simulink model "tren_model"  (Simulink 7.1)
settings: Solver=ode45  StartTime=0.0  StopTime=10.0  RelTol=1e-3
values from neighbouring files (symbols this model uses):
  Ltr1y1 = 12.25    [train_katsayi.m]
  Ltr1y2 = 12.25    [train_katsayi.m]
  Ltr2y1 = 1.25    [train_katsayi.m]
  Ltr2y2 = 1.25    [train_katsayi.m]
  Ltr3y1 = 1.25    [train_katsayi.m]
  Ltr3y2 = 1.25    [train_katsayi.m]
  Vtr = 40    [train_katsayi.m]
settings Model: Creator=DOAN  LastModifiedBy=DOAN

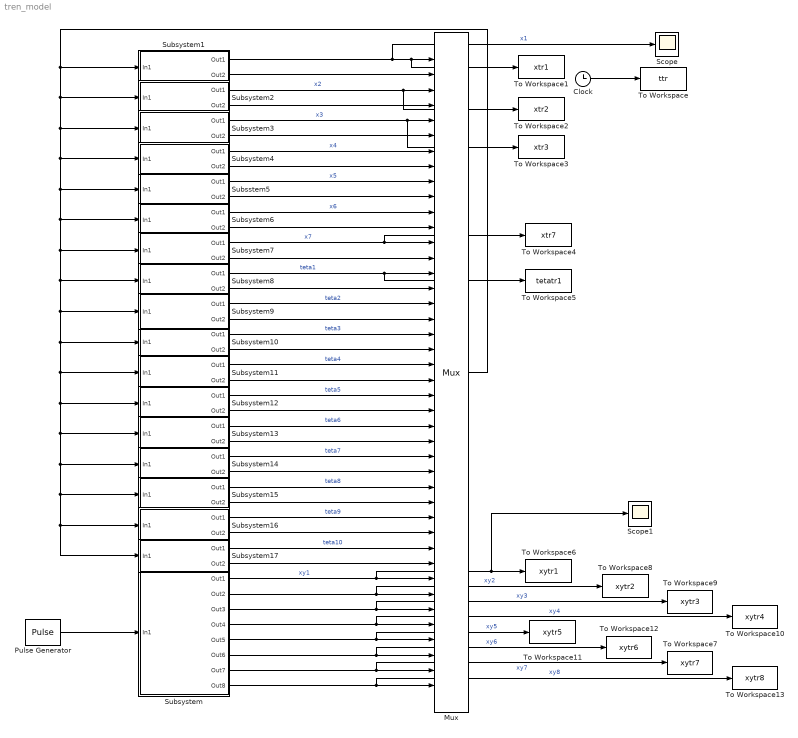
== system tren_model ==
  Clock : Clock
      settings: Decimation=10
  Mux : Mux  Inputs=42
  Pulse Generator : DiscretePulseGenerator  PulseType=Time based  Amplitude=-0.01  Period=0.5  PulseWidth=0.025
  Scope : Scope
      settings: TimeRange=10  YMin=-5e-006  YMax=1.000000000000001e-006
  Scope1 : Scope
      settings: TimeRange=10  YMin=-5e-006  YMax=1.000000000000001e-006
  Subsstem5 : Subsystem
  Subsystem : Subsystem
  Subsystem1 : Subsystem
  Subsystem10 : Subsystem
  Subsystem11 : Subsystem
  Subsystem12 : Subsystem
  Subsystem13 : Subsystem
  Subsystem14 : Subsystem
  Subsystem15 : Subsystem
  Subsystem16 : Subsystem
  Subsystem17 : Subsystem
  Subsystem2 : Subsystem
  Subsystem3 : Subsystem
  Subsystem4 : Subsystem
  Subsystem6 : Subsystem
  Subsystem7 : Subsystem
  Subsystem8 : Subsystem
  Subsystem9 : Subsystem
  To Workspace : ToWorkspace  VariableName=ttr  SampleTime=-1  SaveFormat=Array
  To Workspace1 : ToWorkspace  VariableName=xtr1  SampleTime=-1  SaveFormat=Array
  To Workspace10 : ToWorkspace  VariableName=xytr4  SampleTime=-1  SaveFormat=Array
  To Workspace11 : ToWorkspace  VariableName=xytr5  SampleTime=-1  SaveFormat=Array
  To Workspace12 : ToWorkspace  VariableName=xytr6  SampleTime=-1  SaveFormat=Array
  To Workspace13 : ToWorkspace  VariableName=xytr8  SampleTime=-1  SaveFormat=Array
  To Workspace2 : ToWorkspace  VariableName=xtr2  SampleTime=-1  SaveFormat=Array
  To Workspace3 : ToWorkspace  VariableName=xtr3  SampleTime=-1  SaveFormat=Array
  To Workspace4 : ToWorkspace  VariableName=xtr7  SampleTime=-1  SaveFormat=Array
  To Workspace5 : ToWorkspace  VariableName=tetatr1  SampleTime=-1  SaveFormat=Array
  To Workspace6 : ToWorkspace  VariableName=xytr1  SampleTime=-1  SaveFormat=Array
  To Workspace7 : ToWorkspace  VariableName=xytr7  SampleTime=-1  SaveFormat=Array
  To Workspace8 : ToWorkspace  VariableName=xytr2  SampleTime=-1  SaveFormat=Array
  To Workspace9 : ToWorkspace  VariableName=xytr3  SampleTime=-1  SaveFormat=Array
  wires:
  Mux/1 -> Subsystem17/1(In1), Subsystem16/1(In1), Subsystem15/1(In1), Subsystem14/1(In1), Subsystem13/1(In1), Subsystem12/1(In1), Subsystem11/1(In1), Subsystem10/1(In1), Subsystem9/1(In1), Subsystem8/1(In1), Subsystem7/1(In1), Subsystem6/1(In1), Subsstem5/1(In1), Subsystem4/1(In1), Subsystem3/1(In1), Subsystem2/1(In1), Subsystem1/1(In1)
  Clock/1 -> To Workspace/1
  Pulse Generator/1 -> Subsystem/1(In1)
  Subsystem1/1(Out1) -> Scope/1, Mux/1, To Workspace1/1  "x1"
  Subsystem1/2(Out2) -> Mux/2
  Subsystem2/1(Out1) -> Mux/3, To Workspace2/1  "x2"
  Subsystem2/2(Out2) -> Mux/4
  Subsystem3/1(Out1) -> Mux/5, To Workspace3/1  "x3"
  Subsystem3/2(Out2) -> Mux/6
  Subsystem4/1(Out1) -> Mux/7  "x4"
  Subsystem4/2(Out2) -> Mux/8
  Subsstem5/1(Out1) -> Mux/9  "x5"
  Subsstem5/2(Out2) -> Mux/10
  Subsystem6/1(Out1) -> Mux/11  "x6"
  Subsystem6/2(Out2) -> Mux/12
  Subsystem7/1(Out1) -> Mux/13, To Workspace4/1  "x7"
  Subsystem7/2(Out2) -> Mux/14
  Subsystem8/1(Out1) -> Mux/15, To Workspace5/1  "teta1"
  Subsystem8/2(Out2) -> Mux/16
  Subsystem9/1(Out1) -> Mux/17  "teta2"
  Subsystem9/2(Out2) -> Mux/18
  Subsystem10/1(Out1) -> Mux/19  "teta3"
  Subsystem10/2(Out2) -> Mux/20
  Subsystem11/1(Out1) -> Mux/21  "teta4"
  Subsystem11/2(Out2) -> Mux/22
  Subsystem12/1(Out1) -> Mux/23  "teta5"
  Subsystem12/2(Out2) -> Mux/24
  Subsystem13/1(Out1) -> Mux/25  "teta6"
  Subsystem13/2(Out2) -> Mux/26
  Subsystem14/1(Out1) -> Mux/27  "teta7"
  Subsystem14/2(Out2) -> Mux/28
  Subsystem15/1(Out1) -> Mux/29  "teta8"
  Subsystem15/2(Out2) -> Mux/30
  Subsystem16/1(Out1) -> Mux/31  "teta9"
  Subsystem16/2(Out2) -> Mux/32
  Subsystem17/1(Out1) -> Mux/33  "teta10"
  Subsystem17/2(Out2) -> Mux/34
  Subsystem/1(Out1) -> Mux/35, To Workspace6/1, Scope1/1  "xy1"
  Subsystem/2(Out2) -> Mux/36, To Workspace8/1  "xy2"
  Subsystem/3(Out3) -> Mux/37, To Workspace9/1  "xy3"
  Subsystem/4(Out4) -> Mux/38, To Workspace10/1  "xy4"
  Subsystem/5(Out5) -> Mux/39, To Workspace11/1  "xy5"
  Subsystem/6(Out6) -> Mux/40, To Workspace12/1  "xy6"
  Subsystem/7(Out7) -> Mux/41, To Workspace7/1  "xy7"
  Subsystem/8(Out8) -> Mux/42, To Workspace13/1  "xy8"

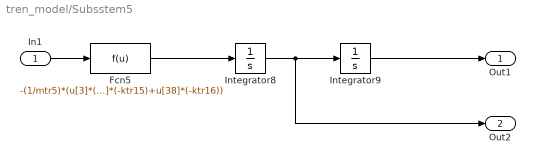
== system tren_model/Subsstem5 ==
  In1 : Inport  OutDataType=sfix(16)  OutScaling=2^0
  Fcn5 : Fcn  Expr=-(1/mtr5)*(u[3]*(-ktr7-ktr8)+u[9]*(ktr7+ktr8+ktr15+ktr16)+u[17]*(ktr7*Ltr2y2+ktr8*Ltr2y2)+u[23]*(ktr7*Ltr2x1-ktr8*Ltr2x2)+u[29]*(-ktr7*Ltr5x1+ktr8*Ltr5x2-ktr15*Ltr5x1+ktr16*Ltr5x2)+u[4]*(-ctr7-ctr8)+u[10]*(ctr7+ctr8)+u[18]*(ctr7*Ltr2y2+ctr8*Ltr2y2)+u[24]*(ctr7*Ltr2x1-ctr8*Ltr2x2)+u[30]*(-ctr7*Ltr5x1+ctr8*Ltr5x2)+u[37]*(-ktr15)+u[38]*(-ktr16))
  Integrator8 : Integrator
  Integrator9 : Integrator
  Out1 : Outport  OutDataType=sfix(16)  OutScaling=2^0
  Out2 : Outport  Port=2  OutDataType=sfix(16)  OutScaling=2^0
  wires:
  Integrator8/1 -> Integrator9/1, Out2/1
  Fcn5/1 -> Integrator8/1
  Integrator9/1 -> Out1/1
  In1/1 -> Fcn5/1

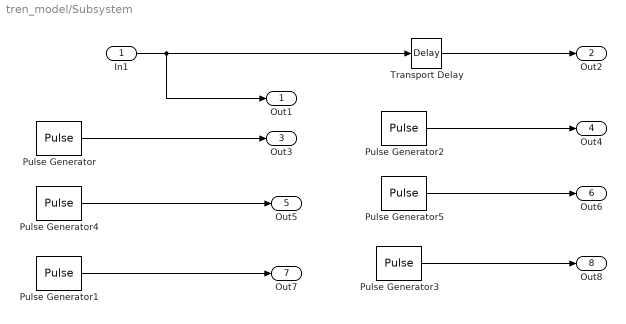
== system tren_model/Subsystem ==
  In1 : Inport  OutDataType=sfix(16)  OutScaling=2^0
  Pulse Generator : DiscretePulseGenerator  PulseType=Time based  Amplitude=-0.01  Period=0.5  PulseWidth=0.025  PhaseDelay=(Ltr2y1+Ltr2y2)/Vtr
  Pulse Generator1 : DiscretePulseGenerator  PulseType=Time based  Amplitude=-0.01  Period=0.5  PulseWidth=0.025  PhaseDelay=(Ltr2y1+Ltr1y1+Ltr1y2+Ltr3y2)/Vtr
  Pulse Generator2 : DiscretePulseGenerator  PulseType=Time based  Amplitude=-0.01  Period=0.5  PulseWidth=0.025  PhaseDelay=(Ltr2y1+Ltr2y2)/Vtr+0.001
  Pulse Generator3 : DiscretePulseGenerator  PulseType=Time based  Amplitude=-0.01  Period=0.5  PulseWidth=0.025  PhaseDelay=(Ltr2y1+Ltr1y1+Ltr1y2+Ltr3y2)/Vtr+0.001
  Pulse Generator4 : DiscretePulseGenerator  PulseType=Time based  Amplitude=-0.01  Period=0.5  PulseWidth=0.025  PhaseDelay=(Ltr2y1+Ltr1y1+Ltr1y2-Ltr3y1)/Vtr
  Pulse Generator5 : DiscretePulseGenerator  PulseType=Time based  Amplitude=-0.01  Period=0.5  PulseWidth=0.025  PhaseDelay=(Ltr2y1+Ltr1y1+Ltr1y2-Ltr3y1)/Vtr+0.001
  Transport Delay : TransportDelay  DelayTime=0.001
  Out1 : Outport  OutDataType=sfix(16)  OutScaling=2^0
  Out2 : Outport  Port=2  OutDataType=sfix(16)  OutScaling=2^0
  Out3 : Outport  Port=3  OutDataType=sfix(16)  OutScaling=2^0
  Out4 : Outport  Port=4  OutDataType=sfix(16)  OutScaling=2^0
  Out5 : Outport  Port=5  OutDataType=sfix(16)  OutScaling=2^0
  Out6 : Outport  Port=6  OutDataType=sfix(16)  OutScaling=2^0
  Out7 : Outport  Port=7  OutDataType=sfix(16)  OutScaling=2^0
  Out8 : Outport  Port=8  OutDataType=sfix(16)  OutScaling=2^0
  wires:
  In1/1 -> Transport Delay/1, Out1/1
  Transport Delay/1 -> Out2/1
  Pulse Generator1/1 -> Out7/1
  Pulse Generator/1 -> Out3/1
  Pulse Generator2/1 -> Out4/1
  Pulse Generator3/1 -> Out8/1
  Pulse Generator4/1 -> Out5/1
  Pulse Generator5/1 -> Out6/1

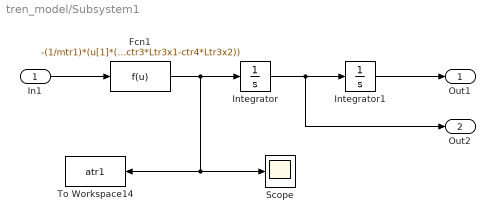
== system tren_model/Subsystem1 ==
  In1 : Inport  OutDataType=sfix(16)  OutScaling=2^0
  Fcn1 : Fcn  Expr=-(1/mtr1)*(u[1]*(ktr1+ktr2+ktr3+ktr4)+u[3]*(-ktr1-ktr2)+u[5]*(-ktr3-ktr4)+u[15]*(ktr1*Ltr1y1+ktr2*Ltr1y1-ktr3*Ltr1y2-ktr4*Ltr1y2)+u[21]*(-ktr1*Ltr1x1+ktr2*Ltr1x2-ktr3*Ltr1x1+ktr4*Ltr1x2)+u[23]*(ktr1*Ltr2x1-ktr2*Ltr2x2)+u[25]*(ktr3*Ltr3x1-ktr4*Ltr3x2)+u[2]*(ctr1+ctr2+ctr3+ctr4)+u[4]*(-ctr1-ctr2)+u[6]*(-ctr3-ctr4)+u[16]*(ctr1*Ltr1y1+ctr2*Ltr1y1-ctr3*Ltr1y2-ctr4*Ltr1y2)+u[22]*(-ctr1*Ltr1x1+ctr2*Ltr1x2-ctr3*Ltr1x1+ctr4*Ltr1x2)+u[24]*(ctr1*Ltr2x1-ctr2*Ltr2x2)+u[26]*(ctr3*Ltr3x1-ctr4*Ltr3x2))
  Integrator : Integrator
  Integrator1 : Integrator
  Scope : Scope
      settings: SaveName=ScopeData2
  To Workspace14 : ToWorkspace  VariableName=atr1  SampleTime=-1  SaveFormat=Array
  Out1 : Outport  OutDataType=sfix(16)  OutScaling=2^0
  Out2 : Outport  Port=2  OutDataType=sfix(16)  OutScaling=2^0
  wires:
  Fcn1/1 -> Integrator/1, Scope/1, To Workspace14/1
  Integrator/1 -> Integrator1/1, Out2/1
  In1/1 -> Fcn1/1
  Integrator1/1 -> Out1/1

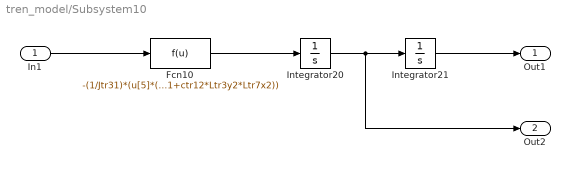
== system tren_model/Subsystem10 ==
  In1 : Inport  OutDataType=sfix(16)  OutScaling=2^0
  Fcn10 : Fcn  Expr=-(1/Jtr31)*(u[5]*(ktr9*Ltr3y1+ktr10*Ltr3y1-ktr11*Ltr3y2-ktr12*Ltr3y2)+u[11]*(-ktr9*Ltr3y1-ktr10*Ltr3y1)+u[13]*(ktr11*Ltr3y2+ktr12*Ltr3y2)+u[19]*(ktr9*Ltr3y1^2+ktr10*Ltr3y1^2+ktr11*Ltr3y2^2+ktr12*Ltr3y2^2)+u[25]*(-ktr9*Ltr3y1*Ltr3x1+ktr10*Ltr3y1*Ltr3x2+ktr11*Ltr3y2*Ltr3x1-ktr12*Ltr3y2*Ltr3x2)+u[31]*(ktr9*Ltr3y1*Ltr6x1-ktr10*Ltr3y1*Ltr6x2)+u[33]*(-ktr11*Ltr3y2*Ltr7x1+ktr12*Ltr3y2*Ltr7x2)+u[6]*(ctr9*Ltr3y1+ctr10*Ltr3y1-ctr11*Ltr3y2-ctr12*Ltr3y2)+u[12]*(-ctr9*Ltr3y1-ctr10*Ltr3y1)+u[14]*(ctr11*Ltr3y2+ctr12*Ltr3y2)+u[20]*(ctr9*Ltr3y1^2+ctr10*Ltr3y1^2+ctr11*Ltr3y2^2+ctr12*Ltr3y2^2)+u[26]*(-ctr9*Ltr3y1*Ltr3x1+ctr10*Ltr3y1*Ltr3x2+ctr11*Ltr3y2*Ltr3x1-ctr12*Ltr3y2*Ltr3x2)+u[32]*(ctr9*Ltr3y1*Ltr6x1-ctr10*Ltr3y1*Ltr6x2)+u[34]*(-ctr11*Ltr3y2*Ltr7x1+ctr12*Ltr3y2*Ltr7x2))
  Integrator20 : Integrator
  Integrator21 : Integrator
  Out1 : Outport  OutDataType=sfix(16)  OutScaling=2^0
  Out2 : Outport  Port=2  OutDataType=sfix(16)  OutScaling=2^0
  wires:
  Integrator20/1 -> Integrator21/1, Out2/1
  Fcn10/1 -> Integrator20/1
  In1/1 -> Fcn10/1
  Integrator21/1 -> Out1/1

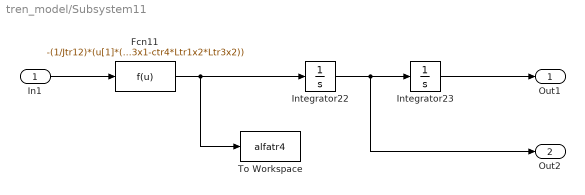
== system tren_model/Subsystem11 ==
  In1 : Inport  OutDataType=sfix(16)  OutScaling=2^0
  Fcn11 : Fcn  Expr=-(1/Jtr12)*(u[1]*(-ktr1*Ltr1x1+ktr2*Ltr1x2-ktr3*Ltr1x1+ktr4*Ltr1x2)+u[3]*(ktr1*Ltr1x1-ktr2*Ltr1x2)+u[5]*(ktr3*Ltr1x1-ktr4*Ltr1x2)+u[15]*(-ktr1*Ltr1x1*Ltr1y1+ktr2*Ltr1x2*Ltr1y1+ktr3*Ltr1x1*Ltr1y2-ktr4*Ltr1x2*Ltr1y2)+u[21]*(ktr1*Ltr1x1^2+ktr2*Ltr1x2^2+ktr3*Ltr1x1^2+ktr4*Ltr1x2^2)+u[23]*(-ktr1*Ltr1x1*Ltr2x1-ktr2*Ltr1x2*Ltr2x2)+u[25]*(-ktr3*Ltr1x1*Ltr3x1-ktr4*Ltr1x2*Ltr3x2)+u[2]*(-ctr1*Ltr1x1+ctr2*Ltr1x2-ctr3*Ltr1x1+ctr4*Ltr1x2)+u[4]*(ctr1*Ltr1x1-ctr2*Ltr1x2)+u[6]*(ctr3*Ltr1x1-ctr4*Ltr1x2)+u[16]*(-ctr1*Ltr1x1*Ltr1y1+ctr2*Ltr1x2*Ltr1y1+ctr3*Ltr1x1*Ltr1y2-ctr4*Ltr1x2*Ltr1y2)+u[22]*(ctr1*Ltr1x1^2+ctr2*Ltr1x2^2+ctr3*Ltr1x1^2+ctr4*Ltr1x2^2)+u[24]*(-ctr1*Ltr1x1*Ltr2x1-ctr2*Ltr1x2*Ltr2x2)+u[26]*(-ctr3*Ltr1x1*Ltr3x1-ctr4*Ltr1x2*Ltr3x2))
  Integrator22 : Integrator
  Integrator23 : Integrator
  To Workspace : ToWorkspace  VariableName=alfatr4  SampleTime=-1  SaveFormat=Array
  Out1 : Outport  OutDataType=sfix(16)  OutScaling=2^0
  Out2 : Outport  Port=2  OutDataType=sfix(16)  OutScaling=2^0
  wires:
  Integrator22/1 -> Integrator23/1, Out2/1
  Fcn11/1 -> Integrator22/1, To Workspace/1
  In1/1 -> Fcn11/1
  Integrator23/1 -> Out1/1

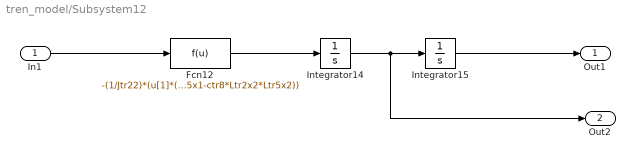
== system tren_model/Subsystem12 ==
  In1 : Inport  OutDataType=sfix(16)  OutScaling=2^0
  Fcn12 : Fcn  Expr=-(1/Jtr22)*(u[1]*(ktr1*Ltr2x1-ktr2*Ltr2x2)+u[3]*(-ktr1*Ltr2x1+ktr2*Ltr2x2-ktr5*Ltr2x1+ktr6*Ltr2x2-ktr7*Ltr2x1+ktr8*Ltr2x2)+u[7]*(ktr5*Ltr2x1-ktr6*Ltr2x2)+u[9]*(ktr7*Ltr2x1-ktr8*Ltr2x2)+u[15]*(ktr1*Ltr2x1*Ltr1y1-ktr2*Ltr2x2*Ltr1y1)+u[17]*(-ktr5*Ltr2x1*Ltr2y1+ktr6*Ltr2x2*Ltr2y1+ktr7*Ltr2x1*Ltr2y2-ktr8*Ltr2x2*Ltr2y2)+u[21]*(-ktr1*Ltr2x1*Ltr1x1-ktr2*Ltr2x2*Ltr1x2)+u[23]*(ktr1*Ltr2x1^2+ktr2*Ltr2x2^2+ktr5*Ltr2x1^2+ktr6*Ltr2x2^2+ktr7*Ltr2x1^2+ktr8*Ltr2x2^2)+u[27]*(-ktr5*Ltr2x1*Ltr4x1-ktr6*Ltr2x2*Ltr4x2)+u[29]*(-ktr7*Ltr2x1*Ltr5x1-ktr8*Ltr2x2*Ltr5x2)+u[2]*(ctr1*Ltr2x1-ctr2*Ltr2x2)+u[4]*(-ctr1*Ltr2x1+ctr2*Ltr2x2-ctr5*Ltr2x1+ctr6*Ltr2x2-ctr7*Ltr2x1+ctr8*Ltr2x2)+u[8]*(ctr5*Ltr2x1-ctr6*Ltr2x2)+u[10]*(ctr7*Ltr2x1-ctr8*Ltr2x2)+u[16]*(ctr1*Ltr2x1*Ltr1y1-ctr2*Ltr2x2*Ltr1y1)+u[18]*(-ctr5*Ltr2x1*Ltr2y1+ctr6*Ltr2x2*Ltr2y1+ctr7*Ltr2x1*Ltr2y2-ctr8*Ltr2x2*Ltr2y2)+u[22]*(-ctr1*Ltr2x1*Ltr1x1-ctr2*Ltr2x2*Ltr1x2)+u[24]*(ctr1*Ltr2x1^2+ctr2*Ltr2x2^2+ctr5*Ltr2x1^2+ctr6*Ltr2x2^2+ctr7*Ltr2x1^2+ctr8*Ltr2x2^2)+u[28]*(-ctr5*Ltr2x1*Ltr4x1-ctr6*Ltr2x2*Ltr4x2)+u[30]*(-ctr7*Ltr2x1*Ltr5x1-ctr8*Ltr2x2*Ltr5x2))
  Integrator14 : Integrator
  Integrator15 : Integrator
  Out1 : Outport  OutDataType=sfix(16)  OutScaling=2^0
  Out2 : Outport  Port=2  OutDataType=sfix(16)  OutScaling=2^0
  wires:
  Integrator14/1 -> Integrator15/1, Out2/1
  Fcn12/1 -> Integrator14/1
  In1/1 -> Fcn12/1
  Integrator15/1 -> Out1/1

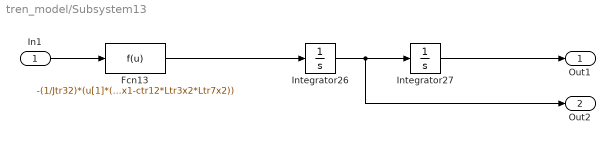
== system tren_model/Subsystem13 ==
  In1 : Inport  OutDataType=sfix(16)  OutScaling=2^0
  Fcn13 : Fcn  Expr=-(1/Jtr32)*(u[1]*(ktr3*Ltr3x1-ktr4*Ltr3x2)+u[5]*(-ktr3*Ltr3x1+ktr4*Ltr3x2-ktr9*Ltr3x1+ktr10*Ltr3x2-ktr11*Ltr3x1+ktr12*Ltr3x2)+u[11]*(ktr9*Ltr3x1-ktr10*Ltr3x2)+u[13]*(ktr11*Ltr3x1-ktr12*Ltr3x2)+u[15]*(-ktr3*Ltr3x1*Ltr1y2+ktr4*Ltr3x2*Ltr1y2)+u[19]*(-ktr9*Ltr3x1*Ltr3y1+ktr10*Ltr3x2*Ltr3y1+ktr11*Ltr3x1*Ltr3y2-ktr12*Ltr3x2*Ltr3y2)+u[21]*(-ktr3*Ltr3x1*Ltr1x1-ktr4*Ltr3x2*Ltr1x2)+u[25]*(ktr3*Ltr3x1^2+ktr4*Ltr3x2^2+ktr9*Ltr3x1^2+ktr10*Ltr3x2^2+ktr11*Ltr3x1^2+ktr12*Ltr3x2^2)+u[31]*(-ktr9*Ltr3x1*Ltr6x1-ktr10*Ltr3x2*Ltr6x2)+u[33]*(-ktr11*Ltr3x1*Ltr7x1-ktr12*Ltr3x2*Ltr7x2)+u[2]*(ctr3*Ltr3x1-ctr4*Ltr3x2)+u[6]*(-ctr3*Ltr3x1+ctr4*Ltr3x2-ctr9*Ltr3x1+ctr10*Ltr3x2-ctr11*Ltr3x1+ctr12*Ltr3x2)+u[12]*(ctr9*Ltr3x1-ctr10*Ltr3x2)+u[14]*(ctr11*Ltr3x1-ctr12*Ltr3x2)+u[16]*(-ctr3*Ltr3x1*Ltr1y2+ctr4*Ltr3x2*Ltr1y2)+u[20]*(-ctr9*Ltr3x1*Ltr3y1+ctr10*Ltr3x2*Ltr3y1+ctr11*Ltr3x1*Ltr3y2-ctr12*Ltr3x2*Ltr3y2)+u[22]*(-ctr3*Ltr3x1*Ltr1x1-ctr4*Ltr3x2*Ltr1x2)+u[26]*(ctr3*Ltr3x1^2+ctr4*Ltr3x2^2+ctr9*Ltr3x1^2+ctr10*Ltr3x2^2+ctr11*Ltr3x1^2+ctr12*Ltr3x2^2)+u[32]*(-ctr9*Ltr3x1*Ltr6x1-ctr10*Ltr3x2*Ltr6x2)+u[34]*(-ctr11*Ltr3x1*Ltr7x1-ctr12*Ltr3x2*Ltr7x2))
  Integrator26 : Integrator
  Integrator27 : Integrator
  Out1 : Outport  OutDataType=sfix(16)  OutScaling=2^0
  Out2 : Outport  Port=2  OutDataType=sfix(16)  OutScaling=2^0
  wires:
  Integrator26/1 -> Integrator27/1, Out2/1
  Fcn13/1 -> Integrator26/1
  In1/1 -> Fcn13/1
  Integrator27/1 -> Out1/1

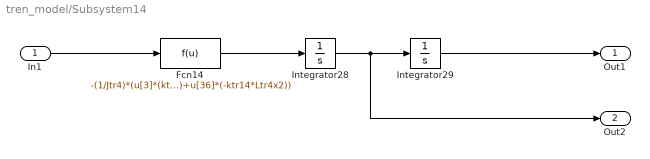
== system tren_model/Subsystem14 ==
  In1 : Inport  OutDataType=sfix(16)  OutScaling=2^0
  Fcn14 : Fcn  Expr=-(1/Jtr4)*(u[3]*(ktr5*Ltr4x1-ktr6*Ltr4x2)+u[7]*(-ktr5*Ltr4x1+ktr6*Ltr4x2-ktr13*Ltr4x1+ktr14*Ltr4x2)+u[17]*(ktr5*Ltr4x1*Ltr2y1-ktr6*Ltr4x2*Ltr2y1)+u[23]*(-ktr5*Ltr4x1*Ltr2x1-ktr6*Ltr4x2*Ltr2x2)+u[27]*(ktr5*Ltr4x1^2+ktr6*Ltr4x2^2+ktr13*Ltr4x1^2+ktr14*Ltr4x2^2)+u[4]*(ctr5*Ltr4x1-ctr6*Ltr4x2)+u[8]*(-ctr5*Ltr4x1+ctr6*Ltr4x2)+u[18]*(ctr5*Ltr4x1*Ltr2y1-ctr6*Ltr4x2*Ltr2y1)+u[24]*(-ctr5*Ltr4x1*Ltr2x1-ctr6*Ltr4x2*Ltr2x2)+u[28]*(ctr5*Ltr4x1^2+ctr6*Ltr4x2^2)+u[35]*(ktr13*Ltr4x1)+u[36]*(-ktr14*Ltr4x2))
  Integrator28 : Integrator
  Integrator29 : Integrator
  Out1 : Outport  OutDataType=sfix(16)  OutScaling=2^0
  Out2 : Outport  Port=2  OutDataType=sfix(16)  OutScaling=2^0
  wires:
  Integrator28/1 -> Integrator29/1, Out2/1
  Fcn14/1 -> Integrator28/1
  In1/1 -> Fcn14/1
  Integrator29/1 -> Out1/1

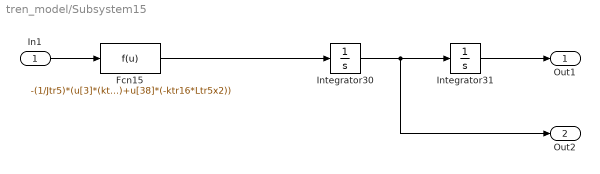
== system tren_model/Subsystem15 ==
  In1 : Inport  OutDataType=sfix(16)  OutScaling=2^0
  Fcn15 : Fcn  Expr=-(1/Jtr5)*(u[3]*(ktr7*Ltr5x1-ktr8*Ltr5x2)+u[9]*(-ktr7*Ltr5x1+ktr8*Ltr5x2-ktr15*Ltr5x1+ktr16*Ltr5x2)+u[17]*(-ktr7*Ltr5x1*Ltr2y2+ktr8*Ltr5x2*Ltr2y2)+u[23]*(-ktr7*Ltr5x1*Ltr2x1-ktr8*Ltr5x2*Ltr2x2)+u[29]*(ktr7*Ltr5x1^2+ktr8*Ltr5x2^2+ktr15*Ltr5x1^2+ktr16*Ltr5x2^2)+u[4]*(ctr7*Ltr5x1-ctr8*Ltr5x2)+u[10]*(-ctr7*Ltr5x1+ctr8*Ltr5x2)+u[18]*(-ctr7*Ltr5x1*Ltr2y2+ctr8*Ltr5x2*Ltr2y2)+u[24]*(-ctr7*Ltr5x1*Ltr2x1-ctr8*Ltr5x2*Ltr2x2)+u[30]*(ctr7*Ltr5x1^2+ctr8*Ltr5x2^2)+u[37]*(ktr15*Ltr5x1)+u[38]*(-ktr16*Ltr5x2))
  Integrator30 : Integrator
  Integrator31 : Integrator
  Out1 : Outport  OutDataType=sfix(16)  OutScaling=2^0
  Out2 : Outport  Port=2  OutDataType=sfix(16)  OutScaling=2^0
  wires:
  Integrator30/1 -> Integrator31/1, Out2/1
  Fcn15/1 -> Integrator30/1
  In1/1 -> Fcn15/1
  Integrator31/1 -> Out1/1

== system tren_model/Subsystem16 ==
  In1 : Inport  OutDataType=sfix(16)  OutScaling=2^0
  Fcn16 : Fcn  Expr=-(1/Jtr6)*(u[5]*(ktr9*Ltr6x1-ktr10*Ltr6x2)+u[11]*(-ktr9*Ltr6x1+ktr10*Ltr6x2-ktr17*Ltr6x1+ktr18*Ltr6x2)+u[19]*(ktr9*Ltr6x1*Ltr3y1-ktr10*Ltr6x2*Ltr3y1)+u[25]*(-ktr9*Ltr6x1*Ltr3x1-ktr10*Ltr6x2*Ltr3x2)+u[31]*(ktr9*Ltr6x1^2+ktr10*Ltr6x2^2+ktr17*Ltr6x1^2+ktr18*Ltr6x2^2)+u[6]*(ctr9*Ltr6x1-ctr10*Ltr6x2)+u[12]*(-ctr9*Ltr6x1+ctr10*Ltr6x2)+u[20]*(ctr9*Ltr6x1*Ltr3y1-ctr10*Ltr6x2*Ltr3y1)+u[26]*(-ctr9*Ltr6x1*Ltr3x1-ctr10*Ltr6x2*Ltr3x2)+u[32]*(ctr9*Ltr6x1^2+ctr10*Ltr6x2^2)+u[39]*(ktr17*Ltr6x1)+u[40]*(-ktr18*Ltr6x2))
  Integrator24 : Integrator
  Integrator25 : Integrator
  Out1 : Outport  OutDataType=sfix(16)  OutScaling=2^0
  Out2 : Outport  Port=2  OutDataType=sfix(16)  OutScaling=2^0
  wires:
  Integrator24/1 -> Integrator25/1, Out2/1
  Fcn16/1 -> Integrator24/1
  In1/1 -> Fcn16/1
  Integrator25/1 -> Out1/1

== system tren_model/Subsystem17 ==
  In1 : Inport  OutDataType=sfix(16)  OutScaling=2^0
  Fcn17 : Fcn  Expr=-(1/Jtr7)*(u[5]*(ktr11*Ltr7x1-ktr12*Ltr7x2)+u[13]*(-ktr11*Ltr7x1+ktr12*Ltr7x2-ktr19*Ltr7x1+ktr20*Ltr7x2)+u[19]*(-ktr11*Ltr7x1*Ltr3y2+ktr12*Ltr7x2*Ltr3y2)+u[25]*(-ktr11*Ltr7x1*Ltr3x1-ktr12*Ltr7x2*Ltr3x2)+u[33]*(ktr11*Ltr7x1^2+ktr12*Ltr7x2^2+ktr19*Ltr7x1^2+ktr20*Ltr7x2^2)+u[6]*(ctr11*Ltr7x1-ctr12*Ltr7x2)+u[14]*(-ctr11*Ltr7x1+ctr12*Ltr7x2)+u[20]*(-ctr11*Ltr7x1*Ltr3y2+ctr12*Ltr7x2*Ltr3y2)+u[26]*(-ctr11*Ltr7x1*Ltr3x1-ctr12*Ltr7x2*Ltr3x2)+u[34]*(ctr11*Ltr7x1^2+ctr12*Ltr7x2^2)+u[41]*(ktr19*Ltr7x1)+u[42]*(-ktr20*Ltr7x2))
  Integrator32 : Integrator
  Integrator33 : Integrator
  Out1 : Outport  OutDataType=sfix(16)  OutScaling=2^0
  Out2 : Outport  Port=2  OutDataType=sfix(16)  OutScaling=2^0
  wires:
  Integrator32/1 -> Integrator33/1, Out2/1
  Fcn17/1 -> Integrator32/1
  In1/1 -> Fcn17/1
  Integrator33/1 -> Out1/1

== system tren_model/Subsystem2 ==
  In1 : Inport  OutDataType=sfix(16)  OutScaling=2^0
  Fcn2 : Fcn  Expr=-(1/mtr2)*(u[1]*(-ktr1-ktr2)+u[3]*(ktr1+ktr2+ktr5+ktr6+ktr7+ktr8)+u[7]*(-ktr5-ktr6)+u[9]*(-ktr7-ktr8)+u[15]*(-ktr1*Ltr1y1-ktr2*Ltr1y1)+u[17]*(ktr5*Ltr2y1+ktr6*Ltr2y1-ktr7*Ltr2y2-ktr8*Ltr2y2)+u[21]*(ktr1*Ltr1x1-ktr2*Ltr1x2)+u[23]*(-ktr1*Ltr2x1+ktr2*Ltr2x2-ktr5*Ltr2x1+ktr6*Ltr2x2-ktr7*Ltr2x1+ktr8*Ltr2x2)+u[27]*(ktr5*Ltr4x1-ktr6*Ltr4x2)+u[29]*(ktr7*Ltr5x1-ktr8*Ltr5x2)+u[2]*(-ctr1-ctr2)+u[4]*(ctr1+ctr2+ctr5+ctr6+ctr7+ctr8)+u[8]*(-ctr5-ctr6)+u[10]*(-ctr7-ctr8)+u[16]*(-ctr1*Ltr1y1-ctr2*Ltr1y1)+u[18]*(ctr5*Ltr2y1+ctr6*Ltr2y1-ctr7*Ltr2y2-ctr8*Ltr2y2)+u[22]*(ctr1*Ltr1x1-ctr2*Ltr1x2)+u[24]*(-ctr1*Ltr2x1+ctr2*Ltr2x2-ctr5*Ltr2x1+ctr6*Ltr2x2-ctr7*Ltr2x1+ctr8*Ltr2x2)+u[28]*(ctr5*Ltr4x1-ctr6*Ltr4x2)+u[30]*(ctr7*Ltr5x1-ctr8*Ltr5x2))
  Integrator2 : Integrator
  Integrator3 : Integrator
  Out1 : Outport  OutDataType=sfix(16)  OutScaling=2^0
  Out2 : Outport  Port=2  OutDataType=sfix(16)  OutScaling=2^0
  wires:
  Fcn2/1 -> Integrator2/1
  Integrator2/1 -> Integrator3/1, Out2/1
  In1/1 -> Fcn2/1
  Integrator3/1 -> Out1/1

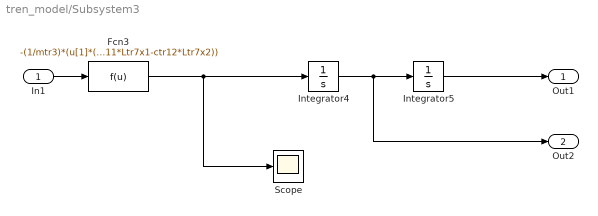
== system tren_model/Subsystem3 ==
  In1 : Inport  OutDataType=sfix(16)  OutScaling=2^0
  Fcn3 : Fcn  Expr=-(1/mtr3)*(u[1]*(-ktr3-ktr4)+u[5]*(ktr3+ktr4+ktr9+ktr10+ktr11+ktr12)+u[11]*(-ktr9-ktr10)+u[13]*(-ktr11-ktr12)+u[15]*(ktr3*Ltr1y2+ktr4*Ltr1y2)+u[19]*(ktr9*Ltr3y1+ktr10*Ltr3y1-ktr11*Ltr3y2-ktr12*Ltr3y2)+u[21]*(ktr3*Ltr1x1-ktr4*Ltr1x2)+u[25]*(-ktr3*Ltr3x1+ktr4*Ltr3x2-ktr9*Ltr3x1+ktr10*Ltr3x2-ktr11*Ltr3x1+ktr12*Ltr3x2)+u[31]*(ktr9*Ltr6x1-ktr10*Ltr6x2)+u[33]*(ktr11*Ltr7x1-ktr12*Ltr7x2)+u[2]*(-ctr3-ctr4)+u[6]*(ctr3+ctr4+ctr9+ctr10+ctr11+ctr12)+u[12]*(-ctr9-ctr10)+u[14]*(-ctr11-ctr12)+u[16]*(ctr3*Ltr1y2+ctr4*Ltr1y2)+u[20]*(ctr9*Ltr3y1+ctr10*Ltr3y1-ctr11*Ltr3y2-ctr12*Ltr3y2)+u[22]*(ctr3*Ltr1x1-ctr4*Ltr1x2)+u[26]*(-ctr3*Ltr3x1+ctr4*Ltr3x2-ctr9*Ltr3x1+ctr10*Ltr3x2-ctr11*Ltr3x1+ctr12*Ltr3x2)+u[32]*(ctr9*Ltr6x1-ctr10*Ltr6x2)+u[34]*(ctr11*Ltr7x1-ctr12*Ltr7x2))
  Integrator4 : Integrator
  Integrator5 : Integrator
  Scope : Scope
      settings: SaveName=ScopeData3
  Out1 : Outport  OutDataType=sfix(16)  OutScaling=2^0
  Out2 : Outport  Port=2  OutDataType=sfix(16)  OutScaling=2^0
  wires:
  Fcn3/1 -> Integrator4/1, Scope/1
  Integrator4/1 -> Integrator5/1, Out2/1
  Integrator5/1 -> Out1/1
  In1/1 -> Fcn3/1

== system tren_model/Subsystem4 ==
  In1 : Inport  OutDataType=sfix(16)  OutScaling=2^0
  Fcn4 : Fcn  Expr=-(1/mtr4)*(u[3]*(-ktr5-ktr6)+u[7]*(ktr5+ktr6+ktr13+ktr14)+u[17]*(-ktr5*Ltr2y1-ktr6*Ltr2y1)+u[23]*(ktr5*Ltr2x1-ktr6*Ltr2x2)+u[27]*(-ktr5*Ltr4x1+ktr6*Ltr4x2-ktr13*Ltr4x1+ktr14*Ltr4x2)+u[4]*(-ctr5-ctr6)+u[8]*(ctr5+ctr6)+u[18]*(-ctr5*Ltr2y1-ctr6*Ltr2y1)+u[24]*(ctr5*Ltr2x1-ctr6*Ltr2x2)+u[28]*(-ctr5*Ltr4x1+ctr6*Ltr4x2)+u[35]*(-ktr13)+u[36]*(-ktr14))
  Integrator6 : Integrator
  Integrator7 : Integrator
  Out1 : Outport  OutDataType=sfix(16)  OutScaling=2^0
  Out2 : Outport  Port=2  OutDataType=sfix(16)  OutScaling=2^0
  wires:
  Fcn4/1 -> Integrator6/1
  Integrator6/1 -> Integrator7/1, Out2/1
  In1/1 -> Fcn4/1
  Integrator7/1 -> Out1/1

== system tren_model/Subsystem6 ==
  In1 : Inport  OutDataType=sfix(16)  OutScaling=2^0
  Fcn6 : Fcn  Expr=-(1/mtr6)*(u[5]*(-ktr9-ktr10)+u[11]*(ktr9+ktr10+ktr17+ktr18)+u[19]*(-ktr9*Ltr3y1-ktr10*Ltr3y1)+u[25]*(ktr9*Ltr3x1-ktr10*Ltr3x2)+u[31]*(-ktr9*Ltr6x1+ktr10*Ltr6x2-ktr17*Ltr6x1+ktr18*Ltr6x2)+u[6]*(-ctr9-ctr10)+u[12]*(ctr9+ctr10)+u[20]*(-ctr9*Ltr3y1-ctr10*Ltr3y1)+u[26]*(ctr9*Ltr3x1-ctr10*Ltr3x2)+u[32]*(-ctr9*Ltr6x1+ctr10*Ltr6x2)+u[39]*(-ktr17)+u[40]*(-ktr18))
  Integrator10 : Integrator
  Integrator11 : Integrator
  Out1 : Outport  OutDataType=sfix(16)  OutScaling=2^0
  Out2 : Outport  Port=2  OutDataType=sfix(16)  OutScaling=2^0
  wires:
  Fcn6/1 -> Integrator10/1
  Integrator10/1 -> Integrator11/1, Out2/1
  In1/1 -> Fcn6/1
  Integrator11/1 -> Out1/1

== system tren_model/Subsystem7 ==
  In1 : Inport  OutDataType=sfix(16)  OutScaling=2^0
  Fcn7 : Fcn  Expr=-(1/mtr7)*(u[5]*(-ktr11-ktr12)+u[13]*(ktr11+ktr12+ktr19+ktr20)+u[19]*(ktr11*Ltr3y2+ktr12*Ltr3y2)+u[25]*(ktr11*Ltr3x1-ktr12*Ltr3x2)+u[33]*(-ktr11*Ltr7x1+ktr12*Ltr7x2-ktr19*Ltr7x1+ktr20*Ltr7x2)+u[6]*(-ctr11-ctr12)+u[14]*(ctr11+ctr12)+u[20]*(ctr11*Ltr3y2+ctr12*Ltr3y2)+u[26]*(ctr11*Ltr3x1-ctr12*Ltr3x2)+u[34]*(-ctr11*Ltr7x1+ctr12*Ltr7x2)+u[41]*(-ktr19)+u[42]*(-ktr20))
  Integrator12 : Integrator
  Integrator13 : Integrator
  Out1 : Outport  OutDataType=sfix(16)  OutScaling=2^0
  Out2 : Outport  Port=2  OutDataType=sfix(16)  OutScaling=2^0
  wires:
  Integrator12/1 -> Integrator13/1, Out2/1
  Fcn7/1 -> Integrator12/1
  In1/1 -> Fcn7/1
  Integrator13/1 -> Out1/1

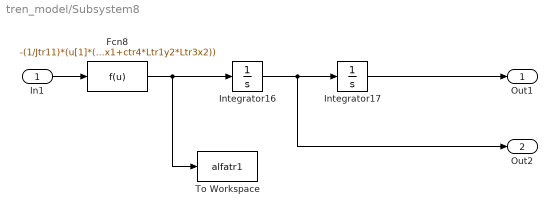
== system tren_model/Subsystem8 ==
  In1 : Inport  OutDataType=sfix(16)  OutScaling=2^0
  Fcn8 : Fcn  Expr=-(1/Jtr11)*(u[1]*(ktr1*Ltr1y1+ktr2*Ltr1y1-ktr3*Ltr1y2-ktr4*Ltr1y2)+u[3]*(-ktr1*Ltr1y1-ktr2*Ltr1y1)+u[5]*(ktr3*Ltr1y2+ktr4*Ltr1y2)+u[15]*(ktr1*Ltr1y1^2+ktr2*Ltr1y1^2+ktr3*Ltr1y2^2+ktr4*Ltr1y2^2)+u[21]*(-ktr1*Ltr1y1*Ltr1x1+ktr2*Ltr1y1*Ltr1x2+ktr3*Ltr1y2*Ltr1x1-ktr4*Ltr1y2*Ltr1x2)+u[23]*(ktr1*Ltr1y1*Ltr2x1-ktr2*Ltr1y1*Ltr2x2)+u[25]*(-ktr3*Ltr1y2*Ltr3x1+ktr4*Ltr1y2*Ltr3x2)+u[2]*(ctr1*Ltr1y1+ctr2*Ltr1y1-ctr3*Ltr1y2-ctr4*Ltr1y2)+u[4]*(-ctr1*Ltr1y1-ctr2*Ltr1y1)+u[6]*(ctr3*Ltr1y2+ctr4*Ltr1y2)+u[16]*(ctr1*Ltr1y1^2+ctr2*Ltr1y1^2+ctr3*Ltr1y2^2+ctr4*Ltr1y2^2)+u[22]*(-ctr1*Ltr1y1*Ltr1x1+ctr2*Ltr1y1*Ltr1x2+ctr3*Ltr1y2*Ltr1x1-ctr4*Ltr1y2*Ltr1x2)+u[24]*(ctr1*Ltr1y1*Ltr2x1-ctr2*Ltr1y1*Ltr2x2)+u[26]*(-ctr3*Ltr1y2*Ltr3x1+ctr4*Ltr1y2*Ltr3x2))
  Integrator16 : Integrator
  Integrator17 : Integrator
  To Workspace : ToWorkspace  VariableName=alfatr1  SampleTime=-1  SaveFormat=Array
  Out1 : Outport  OutDataType=sfix(16)  OutScaling=2^0
  Out2 : Outport  Port=2  OutDataType=sfix(16)  OutScaling=2^0
  wires:
  Integrator16/1 -> Integrator17/1, Out2/1
  Fcn8/1 -> Integrator16/1, To Workspace/1
  In1/1 -> Fcn8/1
  Integrator17/1 -> Out1/1

== system tren_model/Subsystem9 ==
  In1 : Inport  OutDataType=sfix(16)  OutScaling=2^0
  Fcn9 : Fcn  Expr=-(1/Jtr21)*(u[3]*(ktr5*Ltr2y1+ktr6*Ltr2y1-ktr7*Ltr2y2-ktr8*Ltr2y2)+u[7]*(-ktr5*Ltr2y1-ktr6*Ltr2y1)+u[9]*(ktr7*Ltr2y2+ktr8*Ltr2y2)+u[17]*(ktr5*Ltr2y1^2+ktr6*Ltr2y1^2+ktr7*Ltr2y2^2+ktr8*Ltr2y2^2)+u[23]*(-ktr5*Ltr2y1*Ltr2x1+ktr6*Ltr2y1*Ltr2x2+ktr7*Ltr2y2*Ltr2x1-ktr8*Ltr2y2*Ltr2x2)+u[27]*(ktr5*Ltr2y1*Ltr4x1-ktr6*Ltr2y1*Ltr4x2)+u[29]*(-ktr7*Ltr2y2*Ltr5x1+ktr8*Ltr2y2*Ltr5x2)+u[4]*(ctr5*Ltr2y1+ctr6*Ltr2y1-ctr7*Ltr2y2-ctr8*Ltr2y2)+u[8]*(-ctr5*Ltr2y1-ctr6*Ltr2y1)+u[10]*(ctr7*Ltr2y2+ctr8*Ltr2y2)+u[18]*(ctr5*Ltr2y1^2+ctr6*Ltr2y1^2+ctr7*Ltr2y2^2+ctr8*Ltr2y2^2)+u[24]*(-ctr5*Ltr2y1*Ltr2x1+ctr6*Ltr2y1*Ltr2x2+ctr7*Ltr2y2*Ltr2x1-ctr8*Ltr2y2*Ltr2x2)+u[28]*(ctr5*Ltr2y1*Ltr4x1-ctr6*Ltr2y1*Ltr4x2)+u[30]*(-ctr7*Ltr2y2*Ltr5x1+ctr8*Ltr2y2*Ltr5x2))
  Integrator18 : Integrator
  Integrator19 : Integrator
  Out1 : Outport  OutDataType=sfix(16)  OutScaling=2^0
  Out2 : Outport  Port=2  OutDataType=sfix(16)  OutScaling=2^0
  wires:
  Integrator18/1 -> Integrator19/1, Out2/1
  Fcn9/1 -> Integrator18/1
  In1/1 -> Fcn9/1
  Integrator19/1 -> Out1/1
